simulink model "AccGyrXSim"  (R2025b)
settings: Solver=FixedStepDiscrete  StartTime=0.0  StopTime=22  RelTol=1e-3  EnableMultiTasking=on
libraries: mspfiltlib x1
settings Model: Creator=HUB4RT  LastModifiedBy=HUB4RT
settings OptimizationCC: DefaultParameterBehavior=Inlined  EnhancedBackFolding=on  PassReuseOutputArgsAs=Individual arguments  ZeroExternalMemoryAtStartup=off  ZeroInternalMemoryAtStartup=off  MaxStackSize=512  OptimizeBlockOrder=speed  DifferentSizesBufferReuse=on  OptimizationCustomize=off  EfficientTunableParamExpr=on
settings DebuggingCC: ParameterTunabilityLossMsg=error  SFUnexpectedBacktrackingDiag=warning  SFNoUnconditionalDefaultTransitionDiag=warning
settings HardwareCC: ProdBitPerPointer=32.0  ProdBitPerSizeT=32.0  ProdBitPerPtrDiffT=32.0  ProdLargestAtomicInteger=Long  ProdLargestAtomicFloat=Double  ProdWordSize=32.0  ProdLongLongMode=on  ProdHWDeviceType=ARM Compatible->ARM Cortex-M
settings SFSimCC: MATLABDynamicMemAlloc=off
settings RTWCC: SystemTargetFile=ert.tlc  HardwareBoard=STM32H7xx Based (Single-core)  PackageGeneratedCodeAndArtifacts=on  TemplateMakefile=ert_default_tmf  GenerateReport=on  Toolchain=GNU Tools for ARM Embedded Processors  BuildConfiguration=Debug  LaunchReport=on  Description=Embedded Coder
settings CodeAppCC: ForceParamTrailComments=on  IgnoreCustomStorageClasses=off  OperatorAnnotations=on  SimulinkDataObjDesc=on  SFDataObjDesc=on  InsertBlockDesc=on  EnableCustomComments=on
settings ERTTargetCC: ExtModeTransport=3.0  ExtModeStaticAlloc=on  ExtModeStaticAllocSize=2048.0  ExtModeMexFile=ext_xcp  ExtModeIntrfLevel=Level2 - Open  TargetLangStandard=C99 (ISO)  CodeReplacementLibrary=ARM Cortex-M  SupportVariableSizeSignals=on

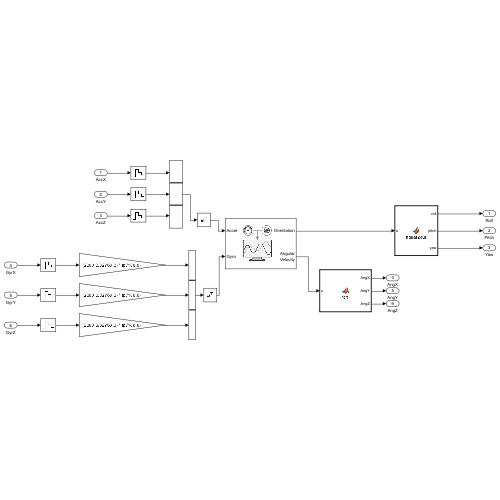
[thumbnail: Simulink's stored preview of the top-level diagram]
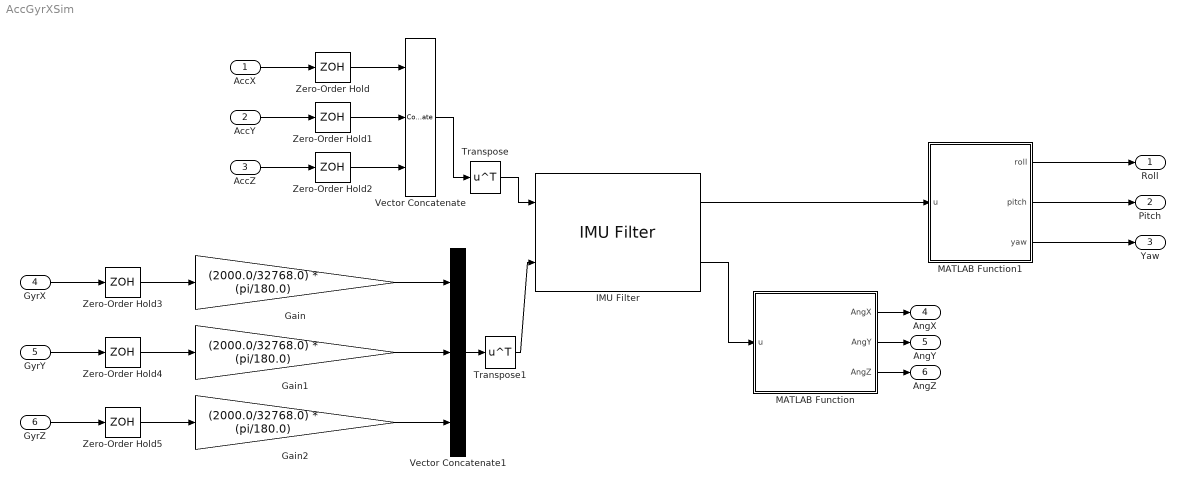
== system AccGyrXSim ==
  AccX : Inport
  AccY : Inport  Port=2
  AccZ : Inport  Port=3
  GyrX : Inport  Port=4
  GyrY : Inport  Port=5
  GyrZ : Inport  Port=6
  Gain : Gain  Gain=(2000.0/32768.0) * (pi/180.0)
  Gain1 : Gain  Gain=(2000.0/32768.0) * (pi/180.0)
  Gain2 : Gain  Gain=(2000.0/32768.0) * (pi/180.0)
  IMU Filter : mspfiltlib/IMU Filter  DispRefFrame=NED  OrientationFormat=quaternion  DecimationFactor=1  InitialProcessNoise=imufilter.defaultProcessNoise  AccelerometerNoise=0.0001924722  GyroscopeNoise=9.1385e-5  GyroscopeDriftNoise=3.0462e-13  LinearAccelerationNoise=0.0096236100000000012  LinearAccelerationDecayFactor=0.5  SimulateUsing=Interpreted execution
  MATLAB Function : MATLAB Function  TreatAsAtomicUnit=on
  MATLAB Function1 : MATLAB Function  TreatAsAtomicUnit=on
  Transpose : Math  Operator=transpose
  Transpose1 : Math  Operator=transpose
  Vector Concatenate : Concatenate  NumInputs=3
  Vector Concatenate1 : Concatenate  NumInputs=3
  Zero-Order Hold{,1..5} (6 alike) : ZeroOrderHold  SampleTime=0.02
  Roll : Outport
  Pitch : Outport  Port=2
  Yaw : Outport  Port=3
  AngX : Outport  Port=4
  AngY : Outport  Port=5
  AngZ : Outport  Port=6
  wires:
  IMU Filter/1 -> MATLAB Function1/1(u)
  MATLAB Function1/1(roll) -> Roll/1
  MATLAB Function1/2(pitch) -> Pitch/1
  MATLAB Function1/3(yaw) -> Yaw/1
  GyrZ/1 -> Zero-Order Hold5/1
  GyrY/1 -> Zero-Order Hold4/1
  Gain2/1 -> Vector Concatenate1/3
  Gain1/1 -> Vector Concatenate1/2
  Gain/1 -> Vector Concatenate1/1
  AccZ/1 -> Zero-Order Hold2/1
  AccY/1 -> Zero-Order Hold1/1
  AccX/1 -> Zero-Order Hold/1
  Transpose/1 -> IMU Filter/1
  Vector Concatenate/1 -> Transpose/1
  Vector Concatenate1/1 -> Transpose1/1
  Transpose1/1 -> IMU Filter/2
  IMU Filter/2 -> MATLAB Function/1(u)
  MATLAB Function/1(AngX) -> AngX/1
  MATLAB Function/2(AngY) -> AngY/1
  MATLAB Function/3(AngZ) -> AngZ/1
  Zero-Order Hold/1 -> Vector Concatenate/1
  Zero-Order Hold1/1 -> Vector Concatenate/2
  Zero-Order Hold2/1 -> Vector Concatenate/3
  Zero-Order Hold5/1 -> Gain2/1
  Zero-Order Hold4/1 -> Gain1/1
  GyrX/1 -> Zero-Order Hold3/1
  Zero-Order Hold3/1 -> Gain/1

== matlab function AccGyrXSim/MATLAB Function ==
  data: u input; AngX output; AngY output; AngZ output
function [AngX,AngY,AngZ] = fcn(u)

y = u;
AngX = y(1);
AngY = y(2);
AngZ = y(3);

== matlab function AccGyrXSim/MATLAB Function1 ==
  data: u input; roll output; pitch output; yaw output
function [roll, pitch, yaw] = hquat2eul(u)

q2 = quaternion(u(:,1), u(:,2), u(:,3), u(:,4));
y = eulerd(q2, "ZYX", "frame");

yaw = y(3);
pitch = y(2);
roll = y(1)-45;

roll  = mod(roll  + 180, 360) - 180;
pitch = mod(pitch + 180, 360) - 180;
yaw   = mod(yaw   + 180, 360) - 180;
